simulink model "grua2"  (Simulink 7.3)
settings: Solver=ode45  StartTime=0.0  StopTime=30  MaxStep=0.001  RelTol=1e-3
undefined symbols (not defined in the file): Bb, Bc, g, K, L, Mb, Mc, U, x10
settings Model: Creator=samsung  LastModifiedBy=samsung
settings DataIOCC: SaveTime=off

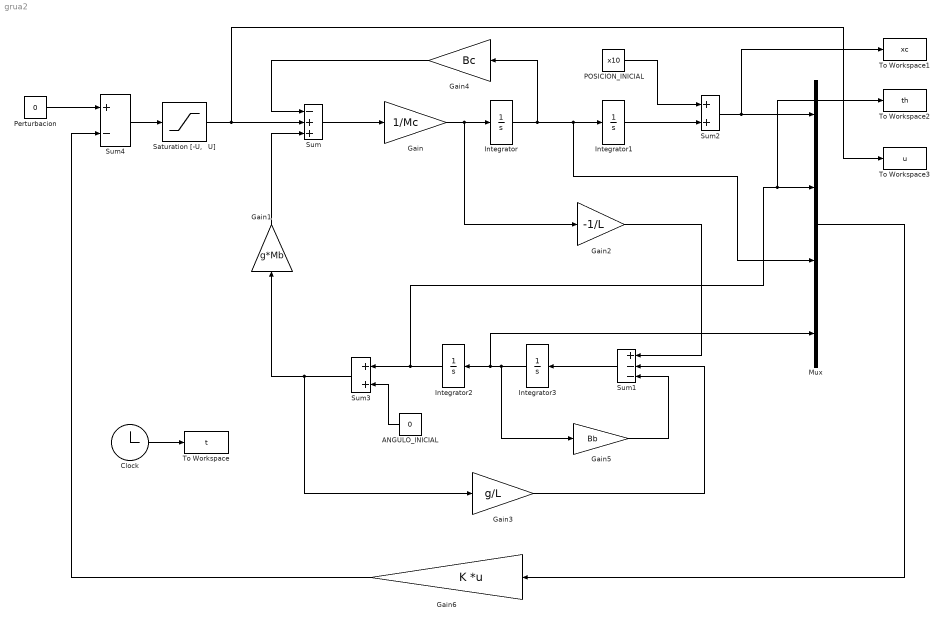
== system grua2 ==
  ANGULO_INICIAL : Constant  Value=0  OutDataType=fixdt(1, 16)  OutScaling=2^0
  Clock : Clock
      settings: Decimation=10
  Gain : Gain  Gain=1/Mc  ParameterDataType=fixdt(1, 16)  ParameterScaling=2^0  OutDataType=fixdt(1, 16)  OutScaling=2^0
  Gain1 : Gain  Gain=g*Mb  ParameterDataType=fixdt(1, 16)  ParameterScaling=2^0  OutDataType=fixdt(1, 16)  OutScaling=2^0
  Gain2 : Gain  Gain=-1/L  ParameterDataType=fixdt(1, 16)  ParameterScaling=2^0  OutDataType=fixdt(1, 16)  OutScaling=2^0
  Gain3 : Gain  Gain=g/L  ParameterDataType=fixdt(1, 16)  ParameterScaling=2^0  OutDataType=fixdt(1, 16)  OutScaling=2^0
  Gain4 : Gain  Gain=Bc  ParameterDataType=fixdt(1, 16)  ParameterScaling=2^0  OutDataType=fixdt(1, 16)  OutScaling=2^0
  Gain5 : Gain  Gain=Bb  ParameterDataType=fixdt(1, 16)  ParameterScaling=2^0  OutDataType=fixdt(1, 16)  OutScaling=2^0
  Gain6 : Gain  Gain=K  Multiplication=Matrix(K*u)  ParameterDataType=fixdt(1, 16)  ParameterScaling=2^0  OutDataType=fixdt(1, 16)  OutScaling=2^0
  Integrator{,1..3} (4 alike) : Integrator
  Mux : Mux
  POSICION_INICIAL : Constant  Value=x10  OutDataType=fixdt(1, 16)  OutScaling=2^0
  Perturbacion : Constant  Value=0  OutDataType=fixdt(1, 16)  OutScaling=2^0
  "Saturation [-U,   U]" : Saturate  UpperLimit=U  LowerLimit=-U  OutDataType=fixdt(1, 16)  OutScaling=2^0
  Sum : Sum  Inputs=-++  OutDataType=fixdt(1, 16)  OutScaling=2^0
  Sum1 : Sum  Inputs=+--  OutDataType=fixdt(1, 16)  OutScaling=2^0
  Sum2 : Sum  OutDataType=fixdt(1, 16)  OutScaling=2^0
  Sum3 : Sum  OutDataType=fixdt(1, 16)  OutScaling=2^0
  Sum4 : Sum  Inputs=+-  OutDataType=fixdt(1, 16)  OutScaling=2^0
  To Workspace : ToWorkspace  VariableName=t  SampleTime=-1  SaveFormat=Array
  To Workspace1 : ToWorkspace  VariableName=xc  SampleTime=-1  SaveFormat=Array
  To Workspace2 : ToWorkspace  VariableName=th  SampleTime=-1  SaveFormat=Array
  To Workspace3 : ToWorkspace  VariableName=u  SampleTime=-1  SaveFormat=Array
  wires:
  Sum4/1 -> "Saturation [-U,   U]"/1
  Gain4/1 -> Sum/1
  "Saturation [-U,   U]"/1 -> Sum/2, To Workspace3/1
  Gain5/1 -> Sum1/3
  Gain3/1 -> Sum1/2
  Gain2/1 -> Sum1/1
  Gain1/1 -> Sum/3
  Sum1/1 -> Integrator3/1
  Integrator3/1 -> Gain5/1, Integrator2/1, Mux/4
  Sum/1 -> Gain/1
  Gain/1 -> Integrator/1, Gain2/1
  Integrator/1 -> Gain4/1, Integrator1/1, Mux/3
  Integrator2/1 -> Sum3/1, Mux/2, To Workspace2/1
  ANGULO_INICIAL/1 -> Sum3/2
  Sum3/1 -> Gain1/1, Gain3/1
  Perturbacion/1 -> Sum4/1
  Gain6/1 -> Sum4/2
  Integrator1/1 -> Sum2/2
  POSICION_INICIAL/1 -> Sum2/1
  Sum2/1 -> Mux/1, To Workspace1/1
  Mux/1 -> Gain6/1
  Clock/1 -> To Workspace/1
